simulink model "d_latch"  (R2018a)
settings: Solver=VariableStepAuto  StartTime=0.0  StopTime=10.0  RelTol=1e-3
settings Model: Creator=Edoardo Debenedetti  LastModifiedBy=Edoardo Debenedetti

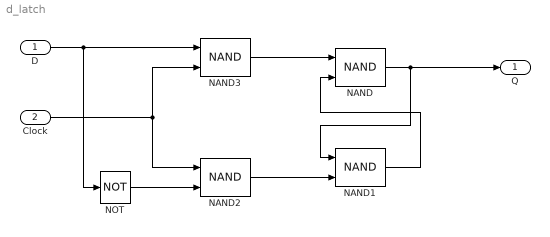
== system d_latch ==
  D : Inport
  Clock : Inport  Port=2
  NAND{,1..3} (4 alike) : Logic  Operator=NAND  IconShape=distinctive  AllPortsSameDT=off  OutDataTypeStr=boolean
  NOT : Logic  Operator=NOT  IconShape=distinctive  AllPortsSameDT=off  OutDataTypeStr=boolean
  Q : Outport
  wires:
  NAND1/1 -> NAND/2
  D/1 -> NAND3/1, NOT/1
  NAND/1 -> NAND1/1, Q/1
  NAND2/1 -> NAND1/2
  Clock/1 -> NAND2/1, NAND3/2
  NOT/1 -> NAND2/2
  NAND3/1 -> NAND/1
